simulink model "Timers"  (R2025a)
settings: Solver=FixedStepDiscrete  StartTime=0  StopTime=1  FixedStep=1e-7  RelTol=1e-3
libraries: simulink_extras x216, simulink x13
(part 3 of 7)

== system Timers/Eg: Normal TImer/Counter ==
  INC : Inport
  TC_RST : Inport  Port=2
  Constant : Constant
  D Flip-Flop{1..7,11} (8 alike) : simulink_extras/Flip Flops/D Flip-Flop
  Demux : Demux  Outputs=8
  Half Adder : Subsystem
      settings: PortSchema="{\"entries\":[{\"content\":{\"sides\":[{\"content\":{\"connectorIds\":[\"In1\"]},\"type\":\"ConnectorPlacement.EquallySpacedRectSide\",\"uuid\":\"d3a7e232-15f2-47a9-a065-9480c81dc57e\"},{\"content\":{\"connectorIds\":[\"Out1\"],\"side\":\"RIGHT\"},\"type\":\"ConnectorPlacement.EquallySpacedRectSide\",\"uuid\":\"e118f150-fee7-4aeb-941e-53c3f02c6791\"},{\"content\":{\"connectorIds\":[\"Out2\"],\"side\":\"TOP\"},\"type\":\"ConnectorPlacement.EquallySpacedRectSide\",\"uuid\":\"6d9038ab-faad-455b-a9c5-8fe0bbf34e51\"},{\"content\":{\"connectorIds\":[\"In2\"],\"side\":\"BOTTOM\"},\"type\":\"ConnectorPlacement.EquallySpacedRectSide\",\"uuid\":\"d09c8d4f-08f3-4c52-88a6-8c6db517fc7a\"}]},\"type\":\"ConnectorPlacement.EquallySpacedConnector\",\"uuid\":\"5bc947ce-f1cd-4957-9186-40c14c78de7d\"}],\"packageUris\":[\"http://schema.mathworks.com/mf0/Connector/R2020b\"],\"version\":\"1.0\"}"
  Half Adder1 : Subsystem
      settings: PortSchema="{\"entries\":[{\"content\":{\"sides\":[{\"content\":{\"connectorIds\":[\"In1\"]},\"type\":\"ConnectorPlacement.EquallySpacedRectSide\",\"uuid\":\"d3a7e232-15f2-47a9-a065-9480c81dc57e\"},{\"content\":{\"connectorIds\":[\"Out1\"],\"side\":\"RIGHT\"},\"type\":\"ConnectorPlacement.EquallySpacedRectSide\",\"uuid\":\"e118f150-fee7-4aeb-941e-53c3f02c6791\"},{\"content\":{\"connectorIds\":[\"Out2\"],\"side\":\"TOP\"},\"type\":\"ConnectorPlacement.EquallySpacedRectSide\",\"uuid\":\"6d9038ab-faad-455b-a9c5-8fe0bbf34e51\"},{\"content\":{\"connectorIds\":[\"In2\"],\"side\":\"BOTTOM\"},\"type\":\"ConnectorPlacement.EquallySpacedRectSide\",\"uuid\":\"d09c8d4f-08f3-4c52-88a6-8c6db517fc7a\"}]},\"type\":\"ConnectorPlacement.EquallySpacedConnector\",\"uuid\":\"5bc947ce-f1cd-4957-9186-40c14c78de7d\"}],\"packageUris\":[\"http://schema.mathworks.com/mf0/Connector/R2020b\"],\"version\":\"1.0\"}"
  Half Adder2 : Subsystem
      settings: PortSchema="{\"entries\":[{\"content\":{\"sides\":[{\"content\":{\"connectorIds\":[\"In1\"]},\"type\":\"ConnectorPlacement.EquallySpacedRectSide\",\"uuid\":\"d3a7e232-15f2-47a9-a065-9480c81dc57e\"},{\"content\":{\"connectorIds\":[\"Out1\"],\"side\":\"RIGHT\"},\"type\":\"ConnectorPlacement.EquallySpacedRectSide\",\"uuid\":\"e118f150-fee7-4aeb-941e-53c3f02c6791\"},{\"content\":{\"connectorIds\":[\"Out2\"],\"side\":\"TOP\"},\"type\":\"ConnectorPlacement.EquallySpacedRectSide\",\"uuid\":\"6d9038ab-faad-455b-a9c5-8fe0bbf34e51\"},{\"content\":{\"connectorIds\":[\"In2\"],\"side\":\"BOTTOM\"},\"type\":\"ConnectorPlacement.EquallySpacedRectSide\",\"uuid\":\"d09c8d4f-08f3-4c52-88a6-8c6db517fc7a\"}]},\"type\":\"ConnectorPlacement.EquallySpacedConnector\",\"uuid\":\"5bc947ce-f1cd-4957-9186-40c14c78de7d\"}],\"packageUris\":[\"http://schema.mathworks.com/mf0/Connector/R2020b\"],\"version\":\"1.0\"}"
  Half Adder3 : Subsystem
      settings: PortSchema="{\"entries\":[{\"content\":{\"sides\":[{\"content\":{\"connectorIds\":[\"In1\"]},\"type\":\"ConnectorPlacement.EquallySpacedRectSide\",\"uuid\":\"d3a7e232-15f2-47a9-a065-9480c81dc57e\"},{\"content\":{\"connectorIds\":[\"Out1\"],\"side\":\"RIGHT\"},\"type\":\"ConnectorPlacement.EquallySpacedRectSide\",\"uuid\":\"e118f150-fee7-4aeb-941e-53c3f02c6791\"},{\"content\":{\"connectorIds\":[\"Out2\"],\"side\":\"TOP\"},\"type\":\"ConnectorPlacement.EquallySpacedRectSide\",\"uuid\":\"6d9038ab-faad-455b-a9c5-8fe0bbf34e51\"},{\"content\":{\"connectorIds\":[\"In2\"],\"side\":\"BOTTOM\"},\"type\":\"ConnectorPlacement.EquallySpacedRectSide\",\"uuid\":\"d09c8d4f-08f3-4c52-88a6-8c6db517fc7a\"}]},\"type\":\"ConnectorPlacement.EquallySpacedConnector\",\"uuid\":\"5bc947ce-f1cd-4957-9186-40c14c78de7d\"}],\"packageUris\":[\"http://schema.mathworks.com/mf0/Connector/R2020b\"],\"version\":\"1.0\"}"
  Half Adder4 : Subsystem
      settings: PortSchema="{\"entries\":[{\"content\":{\"sides\":[{\"content\":{\"connectorIds\":[\"In1\"]},\"type\":\"ConnectorPlacement.EquallySpacedRectSide\",\"uuid\":\"d3a7e232-15f2-47a9-a065-9480c81dc57e\"},{\"content\":{\"connectorIds\":[\"Out1\"],\"side\":\"RIGHT\"},\"type\":\"ConnectorPlacement.EquallySpacedRectSide\",\"uuid\":\"e118f150-fee7-4aeb-941e-53c3f02c6791\"},{\"content\":{\"connectorIds\":[\"Out2\"],\"side\":\"TOP\"},\"type\":\"ConnectorPlacement.EquallySpacedRectSide\",\"uuid\":\"6d9038ab-faad-455b-a9c5-8fe0bbf34e51\"},{\"content\":{\"connectorIds\":[\"In2\"],\"side\":\"BOTTOM\"},\"type\":\"ConnectorPlacement.EquallySpacedRectSide\",\"uuid\":\"d09c8d4f-08f3-4c52-88a6-8c6db517fc7a\"}]},\"type\":\"ConnectorPlacement.EquallySpacedConnector\",\"uuid\":\"5bc947ce-f1cd-4957-9186-40c14c78de7d\"}],\"packageUris\":[\"http://schema.mathworks.com/mf0/Connector/R2020b\"],\"version\":\"1.0\"}"
  Half Adder5 : Subsystem
      settings: PortSchema="{\"entries\":[{\"content\":{\"sides\":[{\"content\":{\"connectorIds\":[\"In1\"]},\"type\":\"ConnectorPlacement.EquallySpacedRectSide\",\"uuid\":\"d3a7e232-15f2-47a9-a065-9480c81dc57e\"},{\"content\":{\"connectorIds\":[\"Out1\"],\"side\":\"RIGHT\"},\"type\":\"ConnectorPlacement.EquallySpacedRectSide\",\"uuid\":\"e118f150-fee7-4aeb-941e-53c3f02c6791\"},{\"content\":{\"connectorIds\":[\"Out2\"],\"side\":\"TOP\"},\"type\":\"ConnectorPlacement.EquallySpacedRectSide\",\"uuid\":\"6d9038ab-faad-455b-a9c5-8fe0bbf34e51\"},{\"content\":{\"connectorIds\":[\"In2\"],\"side\":\"BOTTOM\"},\"type\":\"ConnectorPlacement.EquallySpacedRectSide\",\"uuid\":\"d09c8d4f-08f3-4c52-88a6-8c6db517fc7a\"}]},\"type\":\"ConnectorPlacement.EquallySpacedConnector\",\"uuid\":\"5bc947ce-f1cd-4957-9186-40c14c78de7d\"}],\"packageUris\":[\"http://schema.mathworks.com/mf0/Connector/R2020b\"],\"version\":\"1.0\"}"
  Half Adder6 : Subsystem
      settings: PortSchema="{\"entries\":[{\"content\":{\"sides\":[{\"content\":{\"connectorIds\":[\"In1\"]},\"type\":\"ConnectorPlacement.EquallySpacedRectSide\",\"uuid\":\"d3a7e232-15f2-47a9-a065-9480c81dc57e\"},{\"content\":{\"connectorIds\":[\"Out1\"],\"side\":\"RIGHT\"},\"type\":\"ConnectorPlacement.EquallySpacedRectSide\",\"uuid\":\"e118f150-fee7-4aeb-941e-53c3f02c6791\"},{\"content\":{\"side\":\"TOP\"},\"type\":\"ConnectorPlacement.EquallySpacedRectSide\",\"uuid\":\"6d9038ab-faad-455b-a9c5-8fe0bbf34e51\"},{\"content\":{\"connectorIds\":[\"In2\"],\"side\":\"BOTTOM\"},\"type\":\"ConnectorPlacement.EquallySpacedRectSide\",\"uuid\":\"d09c8d4f-08f3-4c52-88a6-8c6db517fc7a\"}]},\"type\":\"ConnectorPlacement.EquallySpacedConnector\",\"uuid\":\"5bc947ce-f1cd-4957-9186-40c14c78de7d\"}],\"packageUris\":[\"http://schema.mathworks.com/mf0/Connector/R2020b\"],\"version\":\"1.0\"}"
  Half Adder7 : Subsystem
      settings: PortSchema="{\"entries\":[{\"content\":{\"sides\":[{\"content\":{\"connectorIds\":[\"In1\"]},\"type\":\"ConnectorPlacement.EquallySpacedRectSide\",\"uuid\":\"d3a7e232-15f2-47a9-a065-9480c81dc57e\"},{\"content\":{\"connectorIds\":[\"Out1\"],\"side\":\"RIGHT\"},\"type\":\"ConnectorPlacement.EquallySpacedRectSide\",\"uuid\":\"e118f150-fee7-4aeb-941e-53c3f02c6791\"},{\"content\":{\"connectorIds\":[\"Out2\"],\"side\":\"TOP\"},\"type\":\"ConnectorPlacement.EquallySpacedRectSide\",\"uuid\":\"6d9038ab-faad-455b-a9c5-8fe0bbf34e51\"},{\"content\":{\"connectorIds\":[\"In2\"],\"side\":\"BOTTOM\"},\"type\":\"ConnectorPlacement.EquallySpacedRectSide\",\"uuid\":\"d09c8d4f-08f3-4c52-88a6-8c6db517fc7a\"}]},\"type\":\"ConnectorPlacement.EquallySpacedConnector\",\"uuid\":\"5bc947ce-f1cd-4957-9186-40c14c78de7d\"}],\"packageUris\":[\"http://schema.mathworks.com/mf0/Connector/R2020b\"],\"version\":\"1.0\"}"
  Mux1 : Mux  Inputs=8
  Mux2 : Mux  Inputs=8
  NOT : Logic  Operator=NOT  IconShape=distinctive  AllPortsSameDT=off  OutDataTypeStr=boolean
  TC : Outport
  wires:
  TC_RST/1 -> NOT/1
  Mux1/1 -> Demux/1
  Demux/4 -> D Flip-Flop4/1
  Demux/3 -> D Flip-Flop2/1
  Demux/2 -> D Flip-Flop3/1
  Demux/1 -> D Flip-Flop1/1
  Demux/8 -> D Flip-Flop7/1
  Demux/7 -> D Flip-Flop5/1
  Demux/6 -> D Flip-Flop6/1
  Demux/5 -> D Flip-Flop11/1
  INC/1 -> D Flip-Flop2/2, D Flip-Flop3/2, D Flip-Flop1/2, D Flip-Flop4/2, D Flip-Flop11/2, D Flip-Flop6/2, D Flip-Flop5/2, D Flip-Flop7/2
  Constant/1 -> Half Adder7/2("B ")
  Half Adder5/2(Carry) -> Half Adder6/2("B ")
  Half Adder/2(Carry) -> Half Adder1/2("B ")
  Half Adder4/1(Sum) -> Mux1/3
  Half Adder6/1(Sum) -> Mux1/1
  Half Adder5/1(Sum) -> Mux1/2
  Half Adder1/1(Sum) -> Mux1/6
  Half Adder/1(Sum) -> Mux1/7
  Half Adder2/1(Sum) -> Mux1/5
  Half Adder2/2(Carry) -> Half Adder3/2("B ")
  Half Adder3/1(Sum) -> Mux1/4
  Half Adder4/2(Carry) -> Half Adder5/2("B ")
  Half Adder3/2(Carry) -> Half Adder4/2("B ")
  Half Adder1/2(Carry) -> Half Adder2/2("B ")
  Half Adder7/1(Sum) -> Mux1/8
  Half Adder7/2(Carry) -> Half Adder/2("B ")
  D Flip-Flop1/1 -> Mux2/1, Half Adder6/1(A)  "D1"
  D Flip-Flop3/1 -> Mux2/2, Half Adder5/1(A)  "D3"
  D Flip-Flop2/1 -> Mux2/3, Half Adder4/1(A)  "D4"
  D Flip-Flop4/1 -> Mux2/4, Half Adder3/1(A)  "D2"
  D Flip-Flop11/1 -> Mux2/5, Half Adder2/1(A)  "D1"
  D Flip-Flop6/1 -> Mux2/6, Half Adder1/1(A)  "D3"
  D Flip-Flop5/1 -> Mux2/7, Half Adder/1(A)  "D4"
  D Flip-Flop7/1 -> Mux2/8, Half Adder7/1(A)  "D2"
  Mux2/1 -> TC/1
  NOT/1 -> D Flip-Flop2/3, D Flip-Flop1/3, D Flip-Flop3/3, D Flip-Flop4/3, D Flip-Flop11/3, D Flip-Flop6/3, D Flip-Flop5/3, D Flip-Flop7/3

== system Timers/Eg: Normal TImer/TController ==
  TReg : Inport
  StoreTCON : Inport  Port=2
  TF_Clear : Inport  Port=3
  Enable : Inport  Port=4
  Interrupt : Inport  Port=5
  "CLR " : Inport  Port=6
  MCLR : Inport  Port=7
  CLK_IN : Inport  Port=8
  MainCLK : Inport  Port=9
  TC : Inport  Port=10
  AND{,1..3} (4 alike) : Logic  IconShape=distinctive  AllPortsSameDT=off  OutDataTypeStr=boolean
  NOT : Logic  Operator=NOT  IconShape=distinctive  AllPortsSameDT=off  OutDataTypeStr=boolean
  OR1 : Logic  Operator=OR  IconShape=distinctive  AllPortsSameDT=off  OutDataTypeStr=boolean
  OR2 : Logic  Operator=OR  IconShape=distinctive  AllPortsSameDT=off  OutDataTypeStr=boolean
  Prescaler_Controller1 : Subsystem
      settings: PortSchema="{\"entries\":[{\"content\":{\"sides\":[{\"content\":{\"connectorIds\":[\"In1\",\"In2\",\"In3\",\"In4\"]},\"type\":\"ConnectorPlacement.EquallySpacedRectSide\",\"uuid\":\"6170e57a-f155-4328-bd43-dda78d71cb36\"},{\"content\":{\"connectorIds\":[\"In6\",\"Out1\",\"Out2\",\"Out3\"],\"side\":\"RIGHT\"},\"type\":\"ConnectorPlacement.EquallySpacedRectSide\",\"uuid\":\"7c0f968d-cb84-43a5-9c9f-f9604511aa56\"},{\"content\":{\"connectorIds\":[\"In5\"],\"side\":\"TOP\"},\"type\":\"ConnectorPlacement.EquallySpacedRectSide\",\"uuid\":\"1355edcf-182b-4fd1-b160-c0d036cb64ee\"}]},\"type\":\"ConnectorPlacement.EquallySpacedConnector\",\"uuid\":\"78984415-bd5b-43a2-9907-2f223cffd06f\"}],\"packageUris\":[\"http://schema.mathworks.com/mf0/Connector/R2020b\"],\"version\":\"1.0\"}"
  S-R Flip-Flop : simulink_extras/Flip Flops/S-R Flip-Flop  initial_condition=0
  INC : Outport
  TC_RST : Outport  Port=2
  TFlag : Outport  Port=3
  Interrupt vector : Outport  Port=4
  TMR_CLR : Outport  Port=5
  wires:
  "CLR "/1 -> OR2/1
  MCLR/1 -> OR2/2
  OR2/1 -> TMR_CLR/1, Prescaler_Controller1/5("CLR ")
  Interrupt/1 -> AND3/2
  AND3/1 -> Interrupt vector/1
  StoreTCON/1 -> Prescaler_Controller1/3(StoreTCON)
  Prescaler_Controller1/2(TC_RST) -> OR1/1
  Prescaler_Controller1/1(INC) -> AND1/1
  Prescaler_Controller1/3(CLK_Next) -> S-R Flip-Flop/1
  TC/1 -> Prescaler_Controller1/6(TC)
  AND2/1 -> S-R Flip-Flop/2, NOT/1, OR1/2
  S-R Flip-Flop/1 -> TFlag/1, AND3/1
  TReg/1 -> Prescaler_Controller1/1(TReg)
  Enable/1 -> Prescaler_Controller1/2(Enable)
  S-R Flip-Flop/2 -> AND/2
  AND/1 -> Prescaler_Controller1/4(CLK)
  CLK_IN/1 -> AND/1
  OR1/1 -> TC_RST/1
  AND1/1 -> INC/1
  NOT/1 -> AND1/2
  TF_Clear/1 -> AND2/1
  MainCLK/1 -> AND2/2

== system Timers/Eg: Normal TImer/TReg ==
  Data bus : Inport
  Store : Inport  Port=2
  CLK : Inport  Port=3
  CLR : Inport  Port=4
  Demux : Demux  Outputs=8
  Mux : Mux  Inputs=8
  Subsystem1 : Subsystem
  Subsystem2 : Subsystem
  Subsystem3 : Subsystem
  Subsystem4 : Subsystem
  Subsystem5 : Subsystem
  Subsystem6 : Subsystem
  Subsystem7 : Subsystem
  Subsystem8 : Subsystem
  "Q Bus " : Outport
  wires:
  Demux/4 -> Subsystem2/1(Data)
  Mux/1 -> "Q Bus "/1
  Demux/2 -> Subsystem1/1(Data)
  Data bus/1 -> Demux/1
  Subsystem6/1(Q) -> Mux/8
  Store/1 -> Subsystem1/2(Store), Subsystem4/2(Store), Subsystem2/2(Store), Subsystem7/2(Store), Subsystem5/2(Store), Subsystem6/2(Store), Subsystem8/2(Store), Subsystem3/2(Store)
  Demux/5 -> Subsystem7/1(Data)
  Demux/7 -> Subsystem8/1(Data)
  Demux/3 -> Subsystem4/1(Data)
  Subsystem7/1(Q) -> Mux/5
  Demux/6 -> Subsystem5/1(Data)
  Subsystem1/1(Q) -> Mux/2
  Demux/1 -> Subsystem3/1(Data)
  Subsystem3/1(Q) -> Mux/1
  Demux/8 -> Subsystem6/1(Data)
  Subsystem8/1(Q) -> Mux/7
  Subsystem2/1(Q) -> Mux/4
  Subsystem4/1(Q) -> Mux/3
  Subsystem5/1(Q) -> Mux/6
  CLK/1 -> Subsystem1/3(Clock), Subsystem4/3(Clock), Subsystem2/3(Clock), Subsystem7/3(Clock), Subsystem5/3(Clock), Subsystem6/3(Clock), Subsystem8/3(Clock), Subsystem3/3(Clock)
  CLR/1 -> Subsystem8/4(Clear), Subsystem5/4(Clear), Subsystem7/4(Clear), Subsystem2/4(Clear), Subsystem4/4(Clear), Subsystem1/4(Clear), Subsystem3/4(Clear), Subsystem6/4(Clear)

== system Timers/Eg: Normal TImer/Tcon ==
  Data bus : Inport
  Store : Inport  Port=2
  CLK : Inport  Port=3
  CLR : Inport  Port=4
  Demux : Demux  Outputs=8
  Subsystem1 : Subsystem
  Subsystem2 : Subsystem
  Subsystem3 : Subsystem
  Subsystem4 : Subsystem
  Subsystem5 : Subsystem
  Subsystem6 : Subsystem
  Subsystem7 : Subsystem
  Subsystem8 : Subsystem
  TE : Outport
  TAR : Outport  Port=2
  TI : Outport  Port=3
  CLK_Sel : Outport  Port=4
  wires:
  Demux/4 -> Subsystem2/1(Data)
  Demux/2 -> Subsystem1/1(Data)
  Data bus/1 -> Demux/1
  Store/1 -> Subsystem1/2(Store), Subsystem4/2(Store), Subsystem2/2(Store), Subsystem7/2(Store), Subsystem5/2(Store), Subsystem6/2(Store), Subsystem8/2(Store), Subsystem3/2(Store)
  Demux/5 -> Subsystem7/1(Data)
  Demux/7 -> Subsystem8/1(Data)
  Demux/3 -> Subsystem4/1(Data)
  Demux/6 -> Subsystem5/1(Data)
  Subsystem1/1(Q) -> TAR/1
  Demux/1 -> Subsystem3/1(Data)
  Subsystem3/1(Q) -> TE/1
  Demux/8 -> Subsystem6/1(Data)
  Subsystem2/1(Q) -> CLK_Sel/1
  Subsystem4/1(Q) -> TI/1
  CLK/1 -> Subsystem1/3(Clock), Subsystem4/3(Clock), Subsystem2/3(Clock), Subsystem7/3(Clock), Subsystem5/3(Clock), Subsystem6/3(Clock), Subsystem8/3(Clock), Subsystem3/3(Clock)
  CLR/1 -> Subsystem8/4(Clear), Subsystem5/4(Clear), Subsystem7/4(Clear), Subsystem2/4(Clear), Subsystem4/4(Clear), Subsystem1/4(Clear), Subsystem3/4(Clear), Subsystem6/4(Clear)

== system Timers/Eg: PWM Driver+  Prescalar/Counter ==
  INC : Inport
  TC_RST : Inport  Port=2
  Constant : Constant
  D Flip-Flop{1..7,11} (8 alike) : simulink_extras/Flip Flops/D Flip-Flop
  Demux : Demux  Outputs=8
  Half Adder : Subsystem
      settings: PortSchema="{\"entries\":[{\"content\":{\"sides\":[{\"content\":{\"connectorIds\":[\"In1\"]},\"type\":\"ConnectorPlacement.EquallySpacedRectSide\",\"uuid\":\"d3a7e232-15f2-47a9-a065-9480c81dc57e\"},{\"content\":{\"connectorIds\":[\"Out1\"],\"side\":\"RIGHT\"},\"type\":\"ConnectorPlacement.EquallySpacedRectSide\",\"uuid\":\"e118f150-fee7-4aeb-941e-53c3f02c6791\"},{\"content\":{\"connectorIds\":[\"Out2\"],\"side\":\"TOP\"},\"type\":\"ConnectorPlacement.EquallySpacedRectSide\",\"uuid\":\"6d9038ab-faad-455b-a9c5-8fe0bbf34e51\"},{\"content\":{\"connectorIds\":[\"In2\"],\"side\":\"BOTTOM\"},\"type\":\"ConnectorPlacement.EquallySpacedRectSide\",\"uuid\":\"d09c8d4f-08f3-4c52-88a6-8c6db517fc7a\"}]},\"type\":\"ConnectorPlacement.EquallySpacedConnector\",\"uuid\":\"5bc947ce-f1cd-4957-9186-40c14c78de7d\"}],\"packageUris\":[\"http://schema.mathworks.com/mf0/Connector/R2020b\"],\"version\":\"1.0\"}"
  Half Adder1 : Subsystem
      settings: PortSchema="{\"entries\":[{\"content\":{\"sides\":[{\"content\":{\"connectorIds\":[\"In1\"]},\"type\":\"ConnectorPlacement.EquallySpacedRectSide\",\"uuid\":\"d3a7e232-15f2-47a9-a065-9480c81dc57e\"},{\"content\":{\"connectorIds\":[\"Out1\"],\"side\":\"RIGHT\"},\"type\":\"ConnectorPlacement.EquallySpacedRectSide\",\"uuid\":\"e118f150-fee7-4aeb-941e-53c3f02c6791\"},{\"content\":{\"connectorIds\":[\"Out2\"],\"side\":\"TOP\"},\"type\":\"ConnectorPlacement.EquallySpacedRectSide\",\"uuid\":\"6d9038ab-faad-455b-a9c5-8fe0bbf34e51\"},{\"content\":{\"connectorIds\":[\"In2\"],\"side\":\"BOTTOM\"},\"type\":\"ConnectorPlacement.EquallySpacedRectSide\",\"uuid\":\"d09c8d4f-08f3-4c52-88a6-8c6db517fc7a\"}]},\"type\":\"ConnectorPlacement.EquallySpacedConnector\",\"uuid\":\"5bc947ce-f1cd-4957-9186-40c14c78de7d\"}],\"packageUris\":[\"http://schema.mathworks.com/mf0/Connector/R2020b\"],\"version\":\"1.0\"}"
  Half Adder2 : Subsystem
      settings: PortSchema="{\"entries\":[{\"content\":{\"sides\":[{\"content\":{\"connectorIds\":[\"In1\"]},\"type\":\"ConnectorPlacement.EquallySpacedRectSide\",\"uuid\":\"d3a7e232-15f2-47a9-a065-9480c81dc57e\"},{\"content\":{\"connectorIds\":[\"Out1\"],\"side\":\"RIGHT\"},\"type\":\"ConnectorPlacement.EquallySpacedRectSide\",\"uuid\":\"e118f150-fee7-4aeb-941e-53c3f02c6791\"},{\"content\":{\"connectorIds\":[\"Out2\"],\"side\":\"TOP\"},\"type\":\"ConnectorPlacement.EquallySpacedRectSide\",\"uuid\":\"6d9038ab-faad-455b-a9c5-8fe0bbf34e51\"},{\"content\":{\"connectorIds\":[\"In2\"],\"side\":\"BOTTOM\"},\"type\":\"ConnectorPlacement.EquallySpacedRectSide\",\"uuid\":\"d09c8d4f-08f3-4c52-88a6-8c6db517fc7a\"}]},\"type\":\"ConnectorPlacement.EquallySpacedConnector\",\"uuid\":\"5bc947ce-f1cd-4957-9186-40c14c78de7d\"}],\"packageUris\":[\"http://schema.mathworks.com/mf0/Connector/R2020b\"],\"version\":\"1.0\"}"
  Half Adder3 : Subsystem
      settings: PortSchema="{\"entries\":[{\"content\":{\"sides\":[{\"content\":{\"connectorIds\":[\"In1\"]},\"type\":\"ConnectorPlacement.EquallySpacedRectSide\",\"uuid\":\"d3a7e232-15f2-47a9-a065-9480c81dc57e\"},{\"content\":{\"connectorIds\":[\"Out1\"],\"side\":\"RIGHT\"},\"type\":\"ConnectorPlacement.EquallySpacedRectSide\",\"uuid\":\"e118f150-fee7-4aeb-941e-53c3f02c6791\"},{\"content\":{\"connectorIds\":[\"Out2\"],\"side\":\"TOP\"},\"type\":\"ConnectorPlacement.EquallySpacedRectSide\",\"uuid\":\"6d9038ab-faad-455b-a9c5-8fe0bbf34e51\"},{\"content\":{\"connectorIds\":[\"In2\"],\"side\":\"BOTTOM\"},\"type\":\"ConnectorPlacement.EquallySpacedRectSide\",\"uuid\":\"d09c8d4f-08f3-4c52-88a6-8c6db517fc7a\"}]},\"type\":\"ConnectorPlacement.EquallySpacedConnector\",\"uuid\":\"5bc947ce-f1cd-4957-9186-40c14c78de7d\"}],\"packageUris\":[\"http://schema.mathworks.com/mf0/Connector/R2020b\"],\"version\":\"1.0\"}"
  Half Adder4 : Subsystem
      settings: PortSchema="{\"entries\":[{\"content\":{\"sides\":[{\"content\":{\"connectorIds\":[\"In1\"]},\"type\":\"ConnectorPlacement.EquallySpacedRectSide\",\"uuid\":\"d3a7e232-15f2-47a9-a065-9480c81dc57e\"},{\"content\":{\"connectorIds\":[\"Out1\"],\"side\":\"RIGHT\"},\"type\":\"ConnectorPlacement.EquallySpacedRectSide\",\"uuid\":\"e118f150-fee7-4aeb-941e-53c3f02c6791\"},{\"content\":{\"connectorIds\":[\"Out2\"],\"side\":\"TOP\"},\"type\":\"ConnectorPlacement.EquallySpacedRectSide\",\"uuid\":\"6d9038ab-faad-455b-a9c5-8fe0bbf34e51\"},{\"content\":{\"connectorIds\":[\"In2\"],\"side\":\"BOTTOM\"},\"type\":\"ConnectorPlacement.EquallySpacedRectSide\",\"uuid\":\"d09c8d4f-08f3-4c52-88a6-8c6db517fc7a\"}]},\"type\":\"ConnectorPlacement.EquallySpacedConnector\",\"uuid\":\"5bc947ce-f1cd-4957-9186-40c14c78de7d\"}],\"packageUris\":[\"http://schema.mathworks.com/mf0/Connector/R2020b\"],\"version\":\"1.0\"}"
  Half Adder5 : Subsystem
      settings: PortSchema="{\"entries\":[{\"content\":{\"sides\":[{\"content\":{\"connectorIds\":[\"In1\"]},\"type\":\"ConnectorPlacement.EquallySpacedRectSide\",\"uuid\":\"d3a7e232-15f2-47a9-a065-9480c81dc57e\"},{\"content\":{\"connectorIds\":[\"Out1\"],\"side\":\"RIGHT\"},\"type\":\"ConnectorPlacement.EquallySpacedRectSide\",\"uuid\":\"e118f150-fee7-4aeb-941e-53c3f02c6791\"},{\"content\":{\"connectorIds\":[\"Out2\"],\"side\":\"TOP\"},\"type\":\"ConnectorPlacement.EquallySpacedRectSide\",\"uuid\":\"6d9038ab-faad-455b-a9c5-8fe0bbf34e51\"},{\"content\":{\"connectorIds\":[\"In2\"],\"side\":\"BOTTOM\"},\"type\":\"ConnectorPlacement.EquallySpacedRectSide\",\"uuid\":\"d09c8d4f-08f3-4c52-88a6-8c6db517fc7a\"}]},\"type\":\"ConnectorPlacement.EquallySpacedConnector\",\"uuid\":\"5bc947ce-f1cd-4957-9186-40c14c78de7d\"}],\"packageUris\":[\"http://schema.mathworks.com/mf0/Connector/R2020b\"],\"version\":\"1.0\"}"
  Half Adder6 : Subsystem
      settings: PortSchema="{\"entries\":[{\"content\":{\"sides\":[{\"content\":{\"connectorIds\":[\"In1\"]},\"type\":\"ConnectorPlacement.EquallySpacedRectSide\",\"uuid\":\"d3a7e232-15f2-47a9-a065-9480c81dc57e\"},{\"content\":{\"connectorIds\":[\"Out1\"],\"side\":\"RIGHT\"},\"type\":\"ConnectorPlacement.EquallySpacedRectSide\",\"uuid\":\"e118f150-fee7-4aeb-941e-53c3f02c6791\"},{\"content\":{\"side\":\"TOP\"},\"type\":\"ConnectorPlacement.EquallySpacedRectSide\",\"uuid\":\"6d9038ab-faad-455b-a9c5-8fe0bbf34e51\"},{\"content\":{\"connectorIds\":[\"In2\"],\"side\":\"BOTTOM\"},\"type\":\"ConnectorPlacement.EquallySpacedRectSide\",\"uuid\":\"d09c8d4f-08f3-4c52-88a6-8c6db517fc7a\"}]},\"type\":\"ConnectorPlacement.EquallySpacedConnector\",\"uuid\":\"5bc947ce-f1cd-4957-9186-40c14c78de7d\"}],\"packageUris\":[\"http://schema.mathworks.com/mf0/Connector/R2020b\"],\"version\":\"1.0\"}"
  Half Adder7 : Subsystem
      settings: PortSchema="{\"entries\":[{\"content\":{\"sides\":[{\"content\":{\"connectorIds\":[\"In1\"]},\"type\":\"ConnectorPlacement.EquallySpacedRectSide\",\"uuid\":\"d3a7e232-15f2-47a9-a065-9480c81dc57e\"},{\"content\":{\"connectorIds\":[\"Out1\"],\"side\":\"RIGHT\"},\"type\":\"ConnectorPlacement.EquallySpacedRectSide\",\"uuid\":\"e118f150-fee7-4aeb-941e-53c3f02c6791\"},{\"content\":{\"connectorIds\":[\"Out2\"],\"side\":\"TOP\"},\"type\":\"ConnectorPlacement.EquallySpacedRectSide\",\"uuid\":\"6d9038ab-faad-455b-a9c5-8fe0bbf34e51\"},{\"content\":{\"connectorIds\":[\"In2\"],\"side\":\"BOTTOM\"},\"type\":\"ConnectorPlacement.EquallySpacedRectSide\",\"uuid\":\"d09c8d4f-08f3-4c52-88a6-8c6db517fc7a\"}]},\"type\":\"ConnectorPlacement.EquallySpacedConnector\",\"uuid\":\"5bc947ce-f1cd-4957-9186-40c14c78de7d\"}],\"packageUris\":[\"http://schema.mathworks.com/mf0/Connector/R2020b\"],\"version\":\"1.0\"}"
  Mux1 : Mux  Inputs=8
  Mux2 : Mux  Inputs=8
  NOT : Logic  Operator=NOT  IconShape=distinctive  AllPortsSameDT=off  OutDataTypeStr=boolean
  TC : Outport
  wires:
  TC_RST/1 -> NOT/1
  Mux1/1 -> Demux/1
  Demux/4 -> D Flip-Flop4/1
  Demux/3 -> D Flip-Flop2/1
  Demux/2 -> D Flip-Flop3/1
  Demux/1 -> D Flip-Flop1/1
  Demux/8 -> D Flip-Flop7/1
  Demux/7 -> D Flip-Flop5/1
  Demux/6 -> D Flip-Flop6/1
  Demux/5 -> D Flip-Flop11/1
  INC/1 -> D Flip-Flop2/2, D Flip-Flop3/2, D Flip-Flop1/2, D Flip-Flop4/2, D Flip-Flop11/2, D Flip-Flop6/2, D Flip-Flop5/2, D Flip-Flop7/2
  Constant/1 -> Half Adder7/2("B ")
  Half Adder5/2(Carry) -> Half Adder6/2("B ")
  Half Adder/2(Carry) -> Half Adder1/2("B ")
  Half Adder4/1(Sum) -> Mux1/3
  Half Adder6/1(Sum) -> Mux1/1
  Half Adder5/1(Sum) -> Mux1/2
  Half Adder1/1(Sum) -> Mux1/6
  Half Adder/1(Sum) -> Mux1/7
  Half Adder2/1(Sum) -> Mux1/5
  Half Adder2/2(Carry) -> Half Adder3/2("B ")
  Half Adder3/1(Sum) -> Mux1/4
  Half Adder4/2(Carry) -> Half Adder5/2("B ")
  Half Adder3/2(Carry) -> Half Adder4/2("B ")
  Half Adder1/2(Carry) -> Half Adder2/2("B ")
  Half Adder7/1(Sum) -> Mux1/8
  Half Adder7/2(Carry) -> Half Adder/2("B ")
  D Flip-Flop1/1 -> Mux2/1, Half Adder6/1(A)  "D1"
  D Flip-Flop3/1 -> Mux2/2, Half Adder5/1(A)  "D3"
  D Flip-Flop2/1 -> Mux2/3, Half Adder4/1(A)  "D4"
  D Flip-Flop4/1 -> Mux2/4, Half Adder3/1(A)  "D2"
  D Flip-Flop11/1 -> Mux2/5, Half Adder2/1(A)  "D1"
  D Flip-Flop6/1 -> Mux2/6, Half Adder1/1(A)  "D3"
  D Flip-Flop5/1 -> Mux2/7, Half Adder/1(A)  "D4"
  D Flip-Flop7/1 -> Mux2/8, Half Adder7/1(A)  "D2"
  Mux2/1 -> TC/1
  NOT/1 -> D Flip-Flop2/3, D Flip-Flop1/3, D Flip-Flop3/3, D Flip-Flop4/3, D Flip-Flop11/3, D Flip-Flop6/3, D Flip-Flop5/3, D Flip-Flop7/3

== system Timers/Eg: PWM Driver+  Prescalar/Counter1 ==
  INC : Inport
  TC_RST : Inport  Port=2
  Constant : Constant
  D Flip-Flop{1..7,11} (8 alike) : simulink_extras/Flip Flops/D Flip-Flop
  Demux : Demux  Outputs=8
  Half Adder : Subsystem
      settings: PortSchema="{\"entries\":[{\"content\":{\"sides\":[{\"content\":{\"connectorIds\":[\"In1\"]},\"type\":\"ConnectorPlacement.EquallySpacedRectSide\",\"uuid\":\"d3a7e232-15f2-47a9-a065-9480c81dc57e\"},{\"content\":{\"connectorIds\":[\"Out1\"],\"side\":\"RIGHT\"},\"type\":\"ConnectorPlacement.EquallySpacedRectSide\",\"uuid\":\"e118f150-fee7-4aeb-941e-53c3f02c6791\"},{\"content\":{\"connectorIds\":[\"Out2\"],\"side\":\"TOP\"},\"type\":\"ConnectorPlacement.EquallySpacedRectSide\",\"uuid\":\"6d9038ab-faad-455b-a9c5-8fe0bbf34e51\"},{\"content\":{\"connectorIds\":[\"In2\"],\"side\":\"BOTTOM\"},\"type\":\"ConnectorPlacement.EquallySpacedRectSide\",\"uuid\":\"d09c8d4f-08f3-4c52-88a6-8c6db517fc7a\"}]},\"type\":\"ConnectorPlacement.EquallySpacedConnector\",\"uuid\":\"5bc947ce-f1cd-4957-9186-40c14c78de7d\"}],\"packageUris\":[\"http://schema.mathworks.com/mf0/Connector/R2020b\"],\"version\":\"1.0\"}"
  Half Adder1 : Subsystem
      settings: PortSchema="{\"entries\":[{\"content\":{\"sides\":[{\"content\":{\"connectorIds\":[\"In1\"]},\"type\":\"ConnectorPlacement.EquallySpacedRectSide\",\"uuid\":\"d3a7e232-15f2-47a9-a065-9480c81dc57e\"},{\"content\":{\"connectorIds\":[\"Out1\"],\"side\":\"RIGHT\"},\"type\":\"ConnectorPlacement.EquallySpacedRectSide\",\"uuid\":\"e118f150-fee7-4aeb-941e-53c3f02c6791\"},{\"content\":{\"connectorIds\":[\"Out2\"],\"side\":\"TOP\"},\"type\":\"ConnectorPlacement.EquallySpacedRectSide\",\"uuid\":\"6d9038ab-faad-455b-a9c5-8fe0bbf34e51\"},{\"content\":{\"connectorIds\":[\"In2\"],\"side\":\"BOTTOM\"},\"type\":\"ConnectorPlacement.EquallySpacedRectSide\",\"uuid\":\"d09c8d4f-08f3-4c52-88a6-8c6db517fc7a\"}]},\"type\":\"ConnectorPlacement.EquallySpacedConnector\",\"uuid\":\"5bc947ce-f1cd-4957-9186-40c14c78de7d\"}],\"packageUris\":[\"http://schema.mathworks.com/mf0/Connector/R2020b\"],\"version\":\"1.0\"}"
  Half Adder2 : Subsystem
      settings: PortSchema="{\"entries\":[{\"content\":{\"sides\":[{\"content\":{\"connectorIds\":[\"In1\"]},\"type\":\"ConnectorPlacement.EquallySpacedRectSide\",\"uuid\":\"d3a7e232-15f2-47a9-a065-9480c81dc57e\"},{\"content\":{\"connectorIds\":[\"Out1\"],\"side\":\"RIGHT\"},\"type\":\"ConnectorPlacement.EquallySpacedRectSide\",\"uuid\":\"e118f150-fee7-4aeb-941e-53c3f02c6791\"},{\"content\":{\"connectorIds\":[\"Out2\"],\"side\":\"TOP\"},\"type\":\"ConnectorPlacement.EquallySpacedRectSide\",\"uuid\":\"6d9038ab-faad-455b-a9c5-8fe0bbf34e51\"},{\"content\":{\"connectorIds\":[\"In2\"],\"side\":\"BOTTOM\"},\"type\":\"ConnectorPlacement.EquallySpacedRectSide\",\"uuid\":\"d09c8d4f-08f3-4c52-88a6-8c6db517fc7a\"}]},\"type\":\"ConnectorPlacement.EquallySpacedConnector\",\"uuid\":\"5bc947ce-f1cd-4957-9186-40c14c78de7d\"}],\"packageUris\":[\"http://schema.mathworks.com/mf0/Connector/R2020b\"],\"version\":\"1.0\"}"
  Half Adder3 : Subsystem
      settings: PortSchema="{\"entries\":[{\"content\":{\"sides\":[{\"content\":{\"connectorIds\":[\"In1\"]},\"type\":\"ConnectorPlacement.EquallySpacedRectSide\",\"uuid\":\"d3a7e232-15f2-47a9-a065-9480c81dc57e\"},{\"content\":{\"connectorIds\":[\"Out1\"],\"side\":\"RIGHT\"},\"type\":\"ConnectorPlacement.EquallySpacedRectSide\",\"uuid\":\"e118f150-fee7-4aeb-941e-53c3f02c6791\"},{\"content\":{\"connectorIds\":[\"Out2\"],\"side\":\"TOP\"},\"type\":\"ConnectorPlacement.EquallySpacedRectSide\",\"uuid\":\"6d9038ab-faad-455b-a9c5-8fe0bbf34e51\"},{\"content\":{\"connectorIds\":[\"In2\"],\"side\":\"BOTTOM\"},\"type\":\"ConnectorPlacement.EquallySpacedRectSide\",\"uuid\":\"d09c8d4f-08f3-4c52-88a6-8c6db517fc7a\"}]},\"type\":\"ConnectorPlacement.EquallySpacedConnector\",\"uuid\":\"5bc947ce-f1cd-4957-9186-40c14c78de7d\"}],\"packageUris\":[\"http://schema.mathworks.com/mf0/Connector/R2020b\"],\"version\":\"1.0\"}"
  Half Adder4 : Subsystem
      settings: PortSchema="{\"entries\":[{\"content\":{\"sides\":[{\"content\":{\"connectorIds\":[\"In1\"]},\"type\":\"ConnectorPlacement.EquallySpacedRectSide\",\"uuid\":\"d3a7e232-15f2-47a9-a065-9480c81dc57e\"},{\"content\":{\"connectorIds\":[\"Out1\"],\"side\":\"RIGHT\"},\"type\":\"ConnectorPlacement.EquallySpacedRectSide\",\"uuid\":\"e118f150-fee7-4aeb-941e-53c3f02c6791\"},{\"content\":{\"connectorIds\":[\"Out2\"],\"side\":\"TOP\"},\"type\":\"ConnectorPlacement.EquallySpacedRectSide\",\"uuid\":\"6d9038ab-faad-455b-a9c5-8fe0bbf34e51\"},{\"content\":{\"connectorIds\":[\"In2\"],\"side\":\"BOTTOM\"},\"type\":\"ConnectorPlacement.EquallySpacedRectSide\",\"uuid\":\"d09c8d4f-08f3-4c52-88a6-8c6db517fc7a\"}]},\"type\":\"ConnectorPlacement.EquallySpacedConnector\",\"uuid\":\"5bc947ce-f1cd-4957-9186-40c14c78de7d\"}],\"packageUris\":[\"http://schema.mathworks.com/mf0/Connector/R2020b\"],\"version\":\"1.0\"}"
  Half Adder5 : Subsystem
      settings: PortSchema="{\"entries\":[{\"content\":{\"sides\":[{\"content\":{\"connectorIds\":[\"In1\"]},\"type\":\"ConnectorPlacement.EquallySpacedRectSide\",\"uuid\":\"d3a7e232-15f2-47a9-a065-9480c81dc57e\"},{\"content\":{\"connectorIds\":[\"Out1\"],\"side\":\"RIGHT\"},\"type\":\"ConnectorPlacement.EquallySpacedRectSide\",\"uuid\":\"e118f150-fee7-4aeb-941e-53c3f02c6791\"},{\"content\":{\"connectorIds\":[\"Out2\"],\"side\":\"TOP\"},\"type\":\"ConnectorPlacement.EquallySpacedRectSide\",\"uuid\":\"6d9038ab-faad-455b-a9c5-8fe0bbf34e51\"},{\"content\":{\"connectorIds\":[\"In2\"],\"side\":\"BOTTOM\"},\"type\":\"ConnectorPlacement.EquallySpacedRectSide\",\"uuid\":\"d09c8d4f-08f3-4c52-88a6-8c6db517fc7a\"}]},\"type\":\"ConnectorPlacement.EquallySpacedConnector\",\"uuid\":\"5bc947ce-f1cd-4957-9186-40c14c78de7d\"}],\"packageUris\":[\"http://schema.mathworks.com/mf0/Connector/R2020b\"],\"version\":\"1.0\"}"
  Half Adder6 : Subsystem
      settings: PortSchema="{\"entries\":[{\"content\":{\"sides\":[{\"content\":{\"connectorIds\":[\"In1\"]},\"type\":\"ConnectorPlacement.EquallySpacedRectSide\",\"uuid\":\"d3a7e232-15f2-47a9-a065-9480c81dc57e\"},{\"content\":{\"connectorIds\":[\"Out1\"],\"side\":\"RIGHT\"},\"type\":\"ConnectorPlacement.EquallySpacedRectSide\",\"uuid\":\"e118f150-fee7-4aeb-941e-53c3f02c6791\"},{\"content\":{\"side\":\"TOP\"},\"type\":\"ConnectorPlacement.EquallySpacedRectSide\",\"uuid\":\"6d9038ab-faad-455b-a9c5-8fe0bbf34e51\"},{\"content\":{\"connectorIds\":[\"In2\"],\"side\":\"BOTTOM\"},\"type\":\"ConnectorPlacement.EquallySpacedRectSide\",\"uuid\":\"d09c8d4f-08f3-4c52-88a6-8c6db517fc7a\"}]},\"type\":\"ConnectorPlacement.EquallySpacedConnector\",\"uuid\":\"5bc947ce-f1cd-4957-9186-40c14c78de7d\"}],\"packageUris\":[\"http://schema.mathworks.com/mf0/Connector/R2020b\"],\"version\":\"1.0\"}"
  Half Adder7 : Subsystem
      settings: PortSchema="{\"entries\":[{\"content\":{\"sides\":[{\"content\":{\"connectorIds\":[\"In1\"]},\"type\":\"ConnectorPlacement.EquallySpacedRectSide\",\"uuid\":\"d3a7e232-15f2-47a9-a065-9480c81dc57e\"},{\"content\":{\"connectorIds\":[\"Out1\"],\"side\":\"RIGHT\"},\"type\":\"ConnectorPlacement.EquallySpacedRectSide\",\"uuid\":\"e118f150-fee7-4aeb-941e-53c3f02c6791\"},{\"content\":{\"connectorIds\":[\"Out2\"],\"side\":\"TOP\"},\"type\":\"ConnectorPlacement.EquallySpacedRectSide\",\"uuid\":\"6d9038ab-faad-455b-a9c5-8fe0bbf34e51\"},{\"content\":{\"connectorIds\":[\"In2\"],\"side\":\"BOTTOM\"},\"type\":\"ConnectorPlacement.EquallySpacedRectSide\",\"uuid\":\"d09c8d4f-08f3-4c52-88a6-8c6db517fc7a\"}]},\"type\":\"ConnectorPlacement.EquallySpacedConnector\",\"uuid\":\"5bc947ce-f1cd-4957-9186-40c14c78de7d\"}],\"packageUris\":[\"http://schema.mathworks.com/mf0/Connector/R2020b\"],\"version\":\"1.0\"}"
  Mux1 : Mux  Inputs=8
  Mux2 : Mux  Inputs=8
  NOT : Logic  Operator=NOT  IconShape=distinctive  AllPortsSameDT=off  OutDataTypeStr=boolean
  TC : Outport
  wires:
  TC_RST/1 -> NOT/1
  Mux1/1 -> Demux/1
  Demux/4 -> D Flip-Flop4/1
  Demux/3 -> D Flip-Flop2/1
  Demux/2 -> D Flip-Flop3/1
  Demux/1 -> D Flip-Flop1/1
  Demux/8 -> D Flip-Flop7/1
  Demux/7 -> D Flip-Flop5/1
  Demux/6 -> D Flip-Flop6/1
  Demux/5 -> D Flip-Flop11/1
  INC/1 -> D Flip-Flop2/2, D Flip-Flop3/2, D Flip-Flop1/2, D Flip-Flop4/2, D Flip-Flop11/2, D Flip-Flop6/2, D Flip-Flop5/2, D Flip-Flop7/2
  Constant/1 -> Half Adder7/2("B ")
  Half Adder5/2(Carry) -> Half Adder6/2("B ")
  Half Adder/2(Carry) -> Half Adder1/2("B ")
  Half Adder4/1(Sum) -> Mux1/3
  Half Adder6/1(Sum) -> Mux1/1
  Half Adder5/1(Sum) -> Mux1/2
  Half Adder1/1(Sum) -> Mux1/6
  Half Adder/1(Sum) -> Mux1/7
  Half Adder2/1(Sum) -> Mux1/5
  Half Adder2/2(Carry) -> Half Adder3/2("B ")
  Half Adder3/1(Sum) -> Mux1/4
  Half Adder4/2(Carry) -> Half Adder5/2("B ")
  Half Adder3/2(Carry) -> Half Adder4/2("B ")
  Half Adder1/2(Carry) -> Half Adder2/2("B ")
  Half Adder7/1(Sum) -> Mux1/8
  Half Adder7/2(Carry) -> Half Adder/2("B ")
  D Flip-Flop1/1 -> Mux2/1, Half Adder6/1(A)  "D1"
  D Flip-Flop3/1 -> Mux2/2, Half Adder5/1(A)  "D3"
  D Flip-Flop2/1 -> Mux2/3, Half Adder4/1(A)  "D4"
  D Flip-Flop4/1 -> Mux2/4, Half Adder3/1(A)  "D2"
  D Flip-Flop11/1 -> Mux2/5, Half Adder2/1(A)  "D1"
  D Flip-Flop6/1 -> Mux2/6, Half Adder1/1(A)  "D3"
  D Flip-Flop5/1 -> Mux2/7, Half Adder/1(A)  "D4"
  D Flip-Flop7/1 -> Mux2/8, Half Adder7/1(A)  "D2"
  Mux2/1 -> TC/1
  NOT/1 -> D Flip-Flop2/3, D Flip-Flop1/3, D Flip-Flop3/3, D Flip-Flop4/3, D Flip-Flop11/3, D Flip-Flop6/3, D Flip-Flop5/3, D Flip-Flop7/3

== system Timers/Eg: PWM Driver+  Prescalar/Prescaler_Controller1 ==
  TReg : Inport
  "CLR " : Inport  Port=2
  Enable : Inport  Port=3
  StoreTReg : Inport  Port=4
  CLK : Inport  Port=5
  TC : Inport  Port=6
  AND{,1..3} (4 alike) : Logic  IconShape=distinctive  AllPortsSameDT=off  OutDataTypeStr=boolean
  Delay One Step : Delay  DelayLength=1
  Demux : Demux  Outputs=8
  NOR : Logic  Operator=NOR  Inputs=8  IconShape=distinctive  AllPortsSameDT=off  OutDataTypeStr=boolean
  NOT : Logic  Operator=NOT  IconShape=distinctive  AllPortsSameDT=off  OutDataTypeStr=boolean
  NOT1 : Logic  Operator=NOT  IconShape=distinctive  AllPortsSameDT=off  OutDataTypeStr=boolean
  OR : Logic  Operator=OR  Inputs=3  IconShape=distinctive  AllPortsSameDT=off  OutDataTypeStr=boolean
  S-R Flip-Flop : simulink_extras/Flip Flops/S-R Flip-Flop  initial_condition=0
  Scope : Scope
      settings: ActiveDisplayYMinimum=-1  ActiveDisplayYMaximum=1  DataLoggingVariableName=ScopeData2
  XOR : Logic  Operator=XOR  IconShape=distinctive  AllPortsSameDT=off  OutDataTypeStr=boolean
  INC : Outport
  TC_RST : Outport  Port=2
  CLK_Next : Outport  Port=3
  wires:
  TReg/1 -> XOR/1
  Demux/1 -> NOR/1
  TC/1 -> XOR/2
  XOR/1 -> Demux/1
  Demux/2 -> NOR/2
  Demux/3 -> NOR/3
  Demux/4 -> NOR/4
  Demux/5 -> NOR/5
  Demux/6 -> NOR/6
  Demux/7 -> NOR/7
  Demux/8 -> NOR/8
  "CLR "/1 -> OR/3
  NOR/1 -> NOT/1, AND1/1
  Enable/1 -> AND1/2, AND/1
  OR/1 -> Delay One Step/1
  StoreTReg/1 -> OR/1
  AND/1 -> INC/1
  Delay One Step/1 -> AND3/1, TC_RST/1
  AND1/1 -> S-R Flip-Flop/1
  S-R Flip-Flop/1 -> AND2/2
  NOT/1 -> AND2/1
  AND2/1 -> OR/2, Scope/1, CLK_Next/1
  CLK/1 -> NOT1/1, AND/2
  AND3/1 -> S-R Flip-Flop/2
  NOT1/1 -> AND3/2

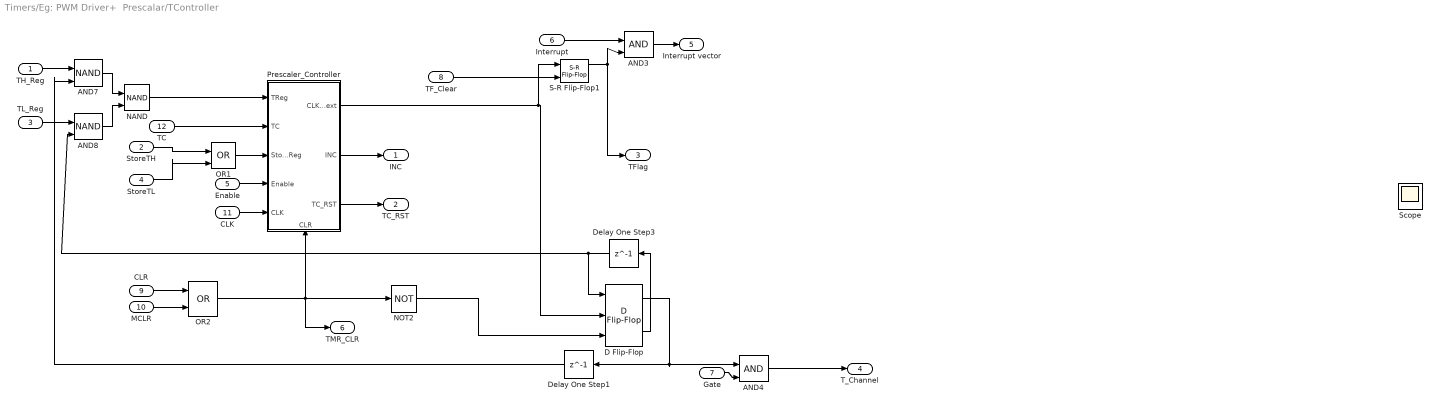
== system Timers/Eg: PWM Driver+  Prescalar/TController ==
  TH_Reg : Inport
  StoreTH : Inport  Port=2
  TL_Reg : Inport  Port=3
  StoreTL : Inport  Port=4
  Enable : Inport  Port=5
  Interrupt : Inport  Port=6
  Gate : Inport  Port=7
  TF_Clear : Inport  Port=8
  "CLR " : Inport  Port=9
  MCLR : Inport  Port=10
  CLK : Inport  Port=11
  TC : Inport  Port=12
  AND3 : Logic  IconShape=distinctive  AllPortsSameDT=off  OutDataTypeStr=boolean
  AND4 : Logic  IconShape=distinctive  AllPortsSameDT=off  OutDataTypeStr=boolean
  AND7 : Logic  Operator=NAND  IconShape=distinctive  AllPortsSameDT=off  OutDataTypeStr=boolean
  AND8 : Logic  Operator=NAND  IconShape=distinctive  AllPortsSameDT=off  OutDataTypeStr=boolean
  D Flip-Flop : simulink_extras/Flip Flops/D Flip-Flop
  Delay One Step1 : Delay  DelayLength=1  SampleTime=1e-5
  Delay One Step3 : Delay  DelayLength=1  SampleTime=1e-5
  NAND : Logic  Operator=NAND  IconShape=distinctive  AllPortsSameDT=off  OutDataTypeStr=boolean
  NOT2 : Logic  Operator=NOT  IconShape=distinctive  AllPortsSameDT=off  OutDataTypeStr=boolean
  OR1 : Logic  Operator=OR  IconShape=distinctive  AllPortsSameDT=off  OutDataTypeStr=boolean
  OR2 : Logic  Operator=OR  IconShape=distinctive  AllPortsSameDT=off  OutDataTypeStr=boolean
  Prescaler_Controller : Subsystem
      settings: PortSchema="{\"entries\":[{\"content\":{\"sides\":[{\"content\":{\"connectorIds\":[\"In1\",\"In2\",\"In3\",\"In4\",\"In5\"]},\"type\":\"ConnectorPlacement.EquallySpacedRectSide\",\"uuid\":\"82b85bc6-964b-49ee-8a4b-3356bfec1aee\"},{\"content\":{\"connectorIds\":[\"Out1\",\"Out2\",\"Out3\"],\"side\":\"RIGHT\"},\"type\":\"ConnectorPlacement.EquallySpacedRectSide\",\"uuid\":\"8c4af632-7d6e-4ec6-a03e-f6796e56340c\"},{\"content\":{\"side\":\"TOP\"},\"type\":\"ConnectorPlacement.EquallySpacedRectSide\",\"uuid\":\"c668d65a-8355-4e30-8ca9-8213ac4eb35c\"},{\"content\":{\"connectorIds\":[\"In6\"],\"side\":\"BOTTOM\"},\"type\":\"ConnectorPlacement.EquallySpacedRectSide\",\"uuid\":\"7e82bb91-fecf-4aec-a971-3b22643d51d5\"}]},\"type\":\"ConnectorPlacement.EquallySpacedConnector\",\"uuid\":\"0a0bd963-09d6-4454-bda2-144190581a2a\"}],\"packageUris\":[\"http://schema.mathworks.com/mf0/Connector/R2020b\"],\"version\":\"1.0\"}"
  S-R Flip-Flop1 : simulink_extras/Flip Flops/S-R Flip-Flop  initial_condition=0
  Scope : Scope
      settings: ActiveDisplayYMinimum=-0.12499999999999997  ActiveDisplayYMaximum=1.125  DataLoggingVariableName=ScopeData5
  INC : Outport
  TC_RST : Outport  Port=2
  TFlag : Outport  Port=3
  T_Channel : Outport  Port=4
  Interrupt vector : Outport  Port=5
  TMR_CLR : Outport  Port=6
  wires:
  "CLR "/1 -> OR2/1
  MCLR/1 -> OR2/2
  Interrupt/1 -> AND3/1
  AND3/1 -> Interrupt vector/1
  Prescaler_Controller/1(CLK_Next) -> S-R Flip-Flop1/1, D Flip-Flop/2
  AND7/1 -> NAND/1
  AND8/1 -> NAND/2
  TH_Reg/1 -> AND7/1
  TL_Reg/1 -> AND8/1
  D Flip-Flop/2 -> Delay One Step3/1
  Delay One Step3/1 -> D Flip-Flop/1, AND8/2
  D Flip-Flop/1 -> Delay One Step1/1, AND4/1
  AND4/1 -> T_Channel/1
  Gate/1 -> AND4/2
  Prescaler_Controller/2(INC) -> INC/1
  OR2/1 -> Prescaler_Controller/6("CLR "), NOT2/1, TMR_CLR/1
  S-R Flip-Flop1/1 -> AND3/2, TFlag/1
  NOT2/1 -> D Flip-Flop/3
  TF_Clear/1 -> S-R Flip-Flop1/2
  Delay One Step1/1 -> AND7/2
  TC/1 -> Prescaler_Controller/2(TC)
  NAND/1 -> Prescaler_Controller/1(TReg)
  OR1/1 -> Prescaler_Controller/3(StoreTReg)
  StoreTH/1 -> OR1/1
  StoreTL/1 -> OR1/2
  Enable/1 -> Prescaler_Controller/4(Enable)
  CLK/1 -> Prescaler_Controller/5(CLK)
  Prescaler_Controller/3(TC_RST) -> TC_RST/1

== system Timers/Eg: PWM Driver+  Prescalar/TH ==
  Data bus : Inport
  Store : Inport  Port=2
  CLK : Inport  Port=3
  CLR : Inport  Port=4
  Demux : Demux  Outputs=8
  Mux : Mux  Inputs=8
  Subsystem1 : Subsystem
  Subsystem2 : Subsystem
  Subsystem3 : Subsystem
  Subsystem4 : Subsystem
  Subsystem5 : Subsystem
  Subsystem6 : Subsystem
  Subsystem7 : Subsystem
  Subsystem8 : Subsystem
  "Q Bus " : Outport
  wires:
  Demux/4 -> Subsystem2/1(Data)
  Mux/1 -> "Q Bus "/1
  Demux/2 -> Subsystem1/1(Data)
  Data bus/1 -> Demux/1
  Subsystem6/1(Q) -> Mux/8
  Store/1 -> Subsystem1/2(Store), Subsystem4/2(Store), Subsystem2/2(Store), Subsystem7/2(Store), Subsystem5/2(Store), Subsystem6/2(Store), Subsystem8/2(Store), Subsystem3/2(Store)
  Demux/5 -> Subsystem7/1(Data)
  Demux/7 -> Subsystem8/1(Data)
  Demux/3 -> Subsystem4/1(Data)
  Subsystem7/1(Q) -> Mux/5
  Demux/6 -> Subsystem5/1(Data)
  Subsystem1/1(Q) -> Mux/2
  Demux/1 -> Subsystem3/1(Data)
  Subsystem3/1(Q) -> Mux/1
  Demux/8 -> Subsystem6/1(Data)
  Subsystem8/1(Q) -> Mux/7
  Subsystem2/1(Q) -> Mux/4
  Subsystem4/1(Q) -> Mux/3
  Subsystem5/1(Q) -> Mux/6
  CLK/1 -> Subsystem1/3(Clock), Subsystem4/3(Clock), Subsystem2/3(Clock), Subsystem7/3(Clock), Subsystem5/3(Clock), Subsystem6/3(Clock), Subsystem8/3(Clock), Subsystem3/3(Clock)
  CLR/1 -> Subsystem8/4(Clear), Subsystem5/4(Clear), Subsystem7/4(Clear), Subsystem2/4(Clear), Subsystem4/4(Clear), Subsystem1/4(Clear), Subsystem3/4(Clear), Subsystem6/4(Clear)

== system Timers/Eg: PWM Driver+  Prescalar/TL ==
  Data bus : Inport
  Store : Inport  Port=2
  CLK : Inport  Port=3
  CLR : Inport  Port=4
  Demux : Demux  Outputs=8
  Mux : Mux  Inputs=8
  Subsystem1 : Subsystem
  Subsystem2 : Subsystem
  Subsystem3 : Subsystem
  Subsystem4 : Subsystem
  Subsystem5 : Subsystem
  Subsystem6 : Subsystem
  Subsystem7 : Subsystem
  Subsystem8 : Subsystem
  "Q Bus " : Outport
  wires:
  Demux/4 -> Subsystem2/1(Data)
  Mux/1 -> "Q Bus "/1
  Demux/2 -> Subsystem1/1(Data)
  Data bus/1 -> Demux/1
  Subsystem6/1(Q) -> Mux/8
  Store/1 -> Subsystem1/2(Store), Subsystem4/2(Store), Subsystem2/2(Store), Subsystem7/2(Store), Subsystem5/2(Store), Subsystem6/2(Store), Subsystem8/2(Store), Subsystem3/2(Store)
  Demux/5 -> Subsystem7/1(Data)
  Demux/7 -> Subsystem8/1(Data)
  Demux/3 -> Subsystem4/1(Data)
  Subsystem7/1(Q) -> Mux/5
  Demux/6 -> Subsystem5/1(Data)
  Subsystem1/1(Q) -> Mux/2
  Demux/1 -> Subsystem3/1(Data)
  Subsystem3/1(Q) -> Mux/1
  Demux/8 -> Subsystem6/1(Data)
  Subsystem8/1(Q) -> Mux/7
  Subsystem2/1(Q) -> Mux/4
  Subsystem4/1(Q) -> Mux/3
  Subsystem5/1(Q) -> Mux/6
  CLK/1 -> Subsystem1/3(Clock), Subsystem4/3(Clock), Subsystem2/3(Clock), Subsystem7/3(Clock), Subsystem5/3(Clock), Subsystem6/3(Clock), Subsystem8/3(Clock), Subsystem3/3(Clock)
  CLR/1 -> Subsystem8/4(Clear), Subsystem5/4(Clear), Subsystem7/4(Clear), Subsystem2/4(Clear), Subsystem4/4(Clear), Subsystem1/4(Clear), Subsystem3/4(Clear), Subsystem6/4(Clear)

== system Timers/Eg: PWM Driver+  Prescalar/TPS ==
  Data bus : Inport
  Store : Inport  Port=2
  CLK : Inport  Port=3
  CLR : Inport  Port=4
  Demux : Demux  Outputs=8
  Mux : Mux  Inputs=8
  Subsystem1 : Subsystem
  Subsystem2 : Subsystem
  Subsystem3 : Subsystem
  Subsystem4 : Subsystem
  Subsystem5 : Subsystem
  Subsystem6 : Subsystem
  Subsystem7 : Subsystem
  Subsystem8 : Subsystem
  "Q Bus " : Outport
  wires:
  Demux/4 -> Subsystem2/1(Data)
  Mux/1 -> "Q Bus "/1
  Demux/2 -> Subsystem1/1(Data)
  Data bus/1 -> Demux/1
  Subsystem6/1(Q) -> Mux/8
  Store/1 -> Subsystem1/2(Store), Subsystem4/2(Store), Subsystem2/2(Store), Subsystem7/2(Store), Subsystem5/2(Store), Subsystem6/2(Store), Subsystem8/2(Store), Subsystem3/2(Store)
  Demux/5 -> Subsystem7/1(Data)
  Demux/7 -> Subsystem8/1(Data)
  Demux/3 -> Subsystem4/1(Data)
  Subsystem7/1(Q) -> Mux/5
  Demux/6 -> Subsystem5/1(Data)
  Subsystem1/1(Q) -> Mux/2
  Demux/1 -> Subsystem3/1(Data)
  Subsystem3/1(Q) -> Mux/1
  Demux/8 -> Subsystem6/1(Data)
  Subsystem8/1(Q) -> Mux/7
  Subsystem2/1(Q) -> Mux/4
  Subsystem4/1(Q) -> Mux/3
  Subsystem5/1(Q) -> Mux/6
  CLK/1 -> Subsystem1/3(Clock), Subsystem4/3(Clock), Subsystem2/3(Clock), Subsystem7/3(Clock), Subsystem5/3(Clock), Subsystem6/3(Clock), Subsystem8/3(Clock), Subsystem3/3(Clock)
  CLR/1 -> Subsystem8/4(Clear), Subsystem5/4(Clear), Subsystem7/4(Clear), Subsystem2/4(Clear), Subsystem4/4(Clear), Subsystem1/4(Clear), Subsystem3/4(Clear), Subsystem6/4(Clear)

== system Timers/Eg: PWM Driver+  Prescalar/Tcon ==
  Data bus : Inport
  Store : Inport  Port=2
  CLK : Inport  Port=3
  CLR : Inport  Port=4
  Demux : Demux  Outputs=8
  Subsystem1 : Subsystem
  Subsystem2 : Subsystem
  Subsystem3 : Subsystem
  Subsystem4 : Subsystem
  Subsystem5 : Subsystem
  Subsystem6 : Subsystem
  Subsystem7 : Subsystem
  Subsystem8 : Subsystem
  TE : Outport
  TAR : Outport  Port=2
  TI : Outport  Port=3
  TG : Outport  Port=4
  wires:
  Demux/4 -> Subsystem2/1(Data)
  Demux/2 -> Subsystem1/1(Data)
  Data bus/1 -> Demux/1
  Store/1 -> Subsystem1/2(Store), Subsystem4/2(Store), Subsystem2/2(Store), Subsystem7/2(Store), Subsystem5/2(Store), Subsystem6/2(Store), Subsystem8/2(Store), Subsystem3/2(Store)
  Demux/5 -> Subsystem7/1(Data)
  Demux/7 -> Subsystem8/1(Data)
  Demux/3 -> Subsystem4/1(Data)
  Demux/6 -> Subsystem5/1(Data)
  Subsystem1/1(Q) -> TAR/1  "Auto Reload"
  Demux/1 -> Subsystem3/1(Data)
  Subsystem3/1(Q) -> TE/1  "Enabled"
  Demux/8 -> Subsystem6/1(Data)
  Subsystem2/1(Q) -> TI/1  "Interrupt"
  Subsystem4/1(Q) -> TG/1  "Gate"
  CLK/1 -> Subsystem1/3(Clock), Subsystem4/3(Clock), Subsystem2/3(Clock), Subsystem7/3(Clock), Subsystem5/3(Clock), Subsystem6/3(Clock), Subsystem8/3(Clock), Subsystem3/3(Clock)
  CLR/1 -> Subsystem8/4(Clear), Subsystem5/4(Clear), Subsystem7/4(Clear), Subsystem2/4(Clear), Subsystem4/4(Clear), Subsystem1/4(Clear), Subsystem3/4(Clear), Subsystem6/4(Clear)
